simulink model "ShootSim"  (R2022a)
settings: Solver=VariableStepAuto  StartTime=0.0  StopTime=10.0  RelTol=1e-3
values from neighbouring files (symbols this model uses):
  A = Bore^2/4    (= 9.0725625e-05)    [Shooting.m]
  k2 = 1/b    (= 2)    [Shooting.m]
  kq = 0.62    [Shooting.m]
  th = V0/(2*beta*kc)    (= 5.98097780479e-12)    [Shooting.m]
  tm = m/b    (= 0.0168)    [Shooting.m]
undefined symbols (not defined in the file or in its folder): k1
settings Model: Creator=JD Herlehy  LastModifiedBy=Eric

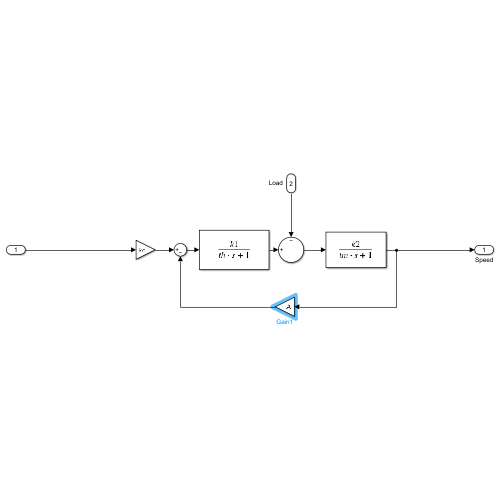
[thumbnail: Simulink's stored preview of the top-level diagram]
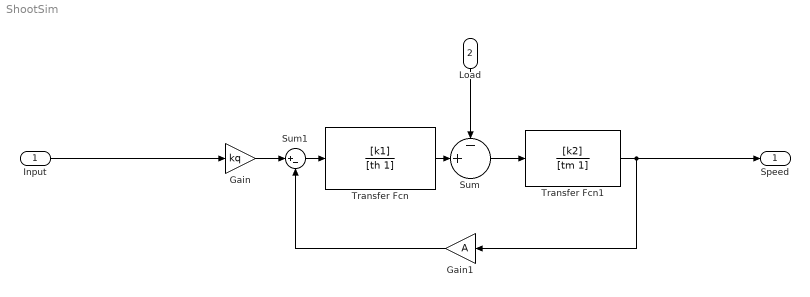
== system ShootSim ==
  Input : Inport
  Load : Inport  Port=2
  Gain : Gain  Gain=kq
  Gain1 : Gain  Gain=A
  Sum : Sum  Inputs=-+|
  Sum1 : Sum  Inputs=|+-
  Transfer Fcn : TransferFcn  Numerator=[k1]  Denominator=[th 1]
  Transfer Fcn1 : TransferFcn  Numerator=[k2]  Denominator=[tm 1]
  Speed : Outport
  wires:
  Gain1/1 -> Sum1/2
  Transfer Fcn/1 -> Sum/2
  Sum1/1 -> Transfer Fcn/1
  Transfer Fcn1/1 -> Speed/1, Gain1/1
  Sum/1 -> Transfer Fcn1/1
  Input/1 -> Gain/1
  Load/1 -> Sum/1
  Gain/1 -> Sum1/1
